simulink model "ExeThree"  (R2017a)
settings: Solver=FixedStepAuto  StartTime=0.0  StopTime=10.0  FixedStep=0.001  RelTol=1e-3
undefined symbols (not defined in the file): c, dF, FGR, m, Tv, vB
settings Model: Creator=22132  LastModifiedBy=22132

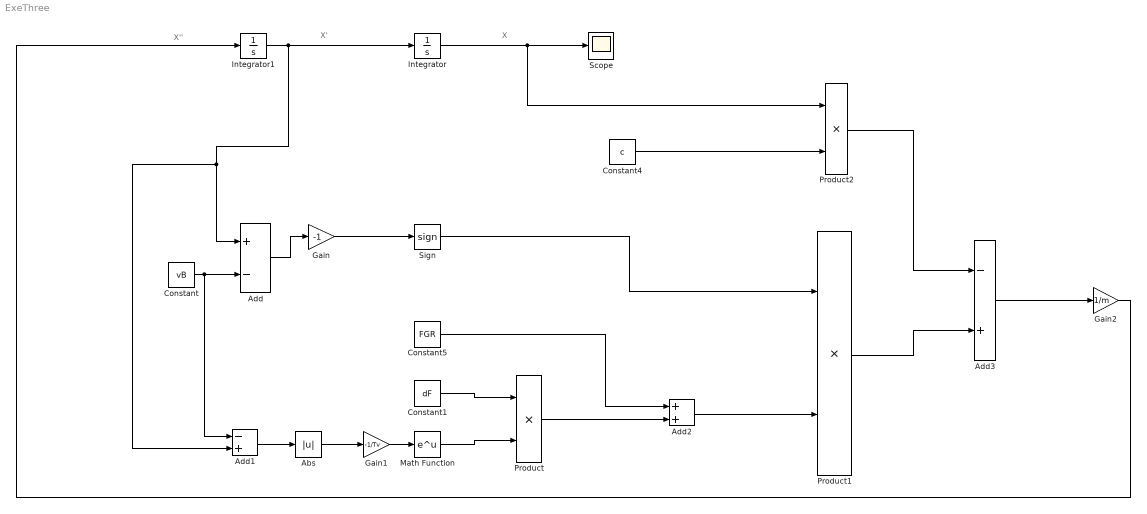
== system ExeThree ==
  note: X''
  note: X'
  note: X
  Abs : Abs
  Add : Sum  Inputs=+-
  Add1 : Sum  Inputs=-+
  Add2 : Sum
  Add3 : Sum  Inputs=-+
  Constant : Constant  Value=vB
  Constant1 : Constant  Value=dF
  Constant4 : Constant  Value=c
  Constant5 : Constant  Value=FGR
  Gain : Gain  Gain=-1
  Gain1 : Gain  Gain=-1/Tv
  Gain2 : Gain  Gain=1/m
  Integrator : Integrator
  Integrator1 : Integrator
  Math Function : Math  SaturateOnIntegerOverflow=on
  Product : Product
  Product1 : Product
  Product2 : Product
  Scope : Scope
  Sign : Signum
  wires:
  Integrator/1 -> Product2/1, Scope/1
  Integrator1/1 -> Add1/2, Add/1, Integrator/1
  Gain/1 -> Sign/1
  Constant/1 -> Add/2, Add1/1
  Add/1 -> Gain/1
  Constant1/1 -> Product/1
  Math Function/1 -> Product/2
  Abs/1 -> Gain1/1
  Add1/1 -> Abs/1
  Gain1/1 -> Math Function/1
  Product/1 -> Add2/2
  Constant5/1 -> Add2/1
  Sign/1 -> Product1/1
  Add2/1 -> Product1/2
  Constant4/1 -> Product2/2
  Product2/1 -> Add3/1
  Product1/1 -> Add3/2
  Add3/1 -> Gain2/1
  Gain2/1 -> Integrator1/1
